simulink model "system_response"  (Simulink 10.1)
settings: Solver=ode45  StartTime=0.0  StopTime=50  MaxStep=.1  MinStep=.05  RelTol=1e-3  EnableMultiTasking=on
settings Model: Creator=ALMOMANI  LastModifiedBy=randai
settings DataIOCC: LimitDataPoints=on
settings OptimizationCC: ExpressionDepthLimit=2147483647
settings DebuggingCC: MultiTaskDSMMsg=warning  MultiTaskCondExecSysMsg=none  FcnCallInpInsideContextMsg=warning  StateNameClashWarn=warning
settings GRTTargetCC: CombineOutputUpdateFcns=on  GRTInterface=off
settings SimscapeCC: SimscapeNormalizeSystem=off
settings ConfigurationSet: Description=SimMechanics 2G

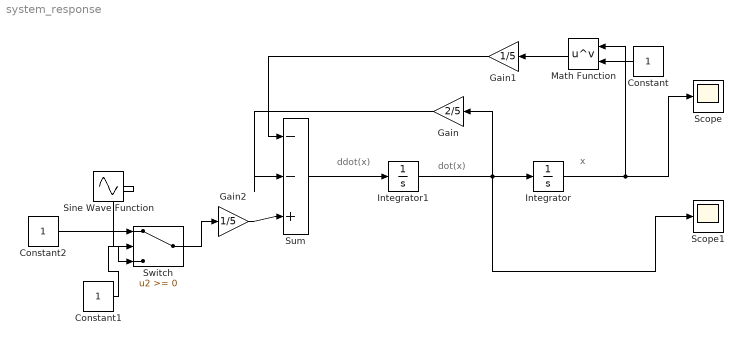
== system system_response ==
  note: x
  note: dot(x)
  note: ddot(x)
  Constant : Constant
  Constant1 : Constant
  Constant2 : Constant
  Gain : Gain  Gain=2/5
  Gain1 : Gain  Gain=1/5
  Gain2 : Gain  Gain=1/5
  Integrator : Integrator  InitialCondition=3
  Integrator1 : Integrator  InitialCondition=-3
  Math Function : Math  Operator=pow  SignedPower=on  SaturateOnIntegerOverflow=on
  Scope : Scope
  Scope1 : Scope
  Sine Wave Function : Sin  Amplitude=3  Frequency=3  SampleTime=0
  Sum : Sum  Inputs=|--+
  Switch : Switch
  wires:
  Integrator/1 -> Math Function/1, Scope/1
  Integrator1/1 -> Scope1/1, Gain/1, Integrator/1
  Constant/1 -> Math Function/2
  Math Function/1 -> Gain1/1
  Sum/1 -> Integrator1/1
  Gain1/1 -> Sum/1
  Gain/1 -> Sum/2
  Sine Wave Function/1 -> Switch/3
  Constant1/1 -> Switch/2
  Switch/1 -> Gain2/1
  Gain2/1 -> Sum/3
  Constant2/1 -> Switch/1
